simulink model "mySimNN"  (R2021a)
settings: Solver=VariableStepAuto  StartTime=0.0  StopTime=30  MaxStep=1e-3  RelTol=1e-3  EnableMultiTasking=on
values from neighbouring files (symbols this model uses):
  K2 = place(A2, B2, eigs)    [linearizedController.m]
undefined symbols (not defined in the file or in its folder): sigbuilder_block
libraries: simulink x2, deeplib x1
settings Model: Creator=The MathWorks, Inc.  LastModifiedBy=danielpusicha
settings SolverCC: AlgebraicLoopSolver=LineSearch  MinimalZcImpactIntegration=on
settings DataIOCC: LimitDataPoints=on  SaveFormat=Structure  ReturnWorkspaceOutputs=off
settings OptimizationCC: LifeSpan=inf
settings DebuggingCC: AlgebraicLoopMsg=none  UnderspecifiedInitializationDetection=Classic  MergeDetectMultiDrivingBlocksExec=none  SolverPrmCheckMsg=warning  AllowSymbolicDim=off  StateNameClashWarn=warning  SFUnexpectedBacktrackingDiag=warning  SFNoUnconditionalDefaultTransitionDiag=warning  SFExecutionAtInitializationDiag=none  SFMachineParentedDataDiag=warning  ArithmeticOperatorsInVariantConditions=warning
settings HardwareCC: ProdBitPerPointer=32  ProdBitPerSizeT=32  ProdBitPerPtrDiffT=32  ProdLargestAtomicFloat=None  ProdIntDivRoundTo=Undefined  ProdEndianess=Unspecified  ProdWordSize=32  ProdHWDeviceType=32-bit Generic
settings ModelReferenceCC: PropagateSignalLabelsOutOfModel=off
settings SFSimCC: SimUseLocalCustomCode=off  CustomCodeUndefinedFunction=UseInterfaceOnly
settings RTWCC: RTWUseLocalCustomCode=off
settings CodeAppCC: StateflowObjectComments=on
settings GRTTargetCC: TargetLangStandard=C89/C90 (ANSI)
settings ConfigComp: CovMetricSettings=dw  CovSaveCumulativeToWorkspaceVar=on  CovSaveSingleToWorkspaceVar=on  CovExternalEMLEnable=off  CovSFcnEnable=off
settings SimscapeCC: SimscapeNormalizeSystem=off
settings ConfigurationSet: Description=SimMechanics 2G
settings ExplorerConfigSet: InternalSimMechanicsExplorerSettings="<ExplorerConfiguration><canonicalview>default</canonicalview><AnimationSetting><BasePlaybackSpeed>1.0</BasePlaybackSpeed><PlaybackSpeedFactor>1.0</PlaybackSpeedFactor></AnimationSetting><TilePanel><TileInfo><Tiles Columns=\"1\" Count=\"1\" Rows=\"1\"><Column Left=\"2\" Weight=\"1\"/><Column Left=\"1552\"/><Row Top=\"2\" Weight=\"1\"/><Row Top=\"932\"/><Tile Height=\"1\" Width=\"1\" X=\"0\" Y=\"0\"/></Tiles></TileInfo><SceneInfo><SceneViewer><BGColor><R>0.60000002384185791</R><G>0.60000002384185791</G><B>0.60000002384185791</B></BGColor><Camera><Position><X>0.027865189060748197</X><Y>-2.5719092456962986</Y><Z>0.23157896538506753</Z></Position><Center><X>0.62659712312732463</X><Y>-0.46110119691712204</Y><Z>0.22087365386473376</Z></Center><Up><X>-0.0079438354874226333</X><Y>0.0073246425924307582</Y><Z>0.99994162084025784</Z></Up><Left>-0.24533778208815546</Left><Right>0.24533778208815546</Right><Bottom>-0.79734779727023208</Bottom><Top>0.79734779727023208</Top></Camera></SceneViewer></SceneInfo></TilePanel></ExplorerConfiguration>"

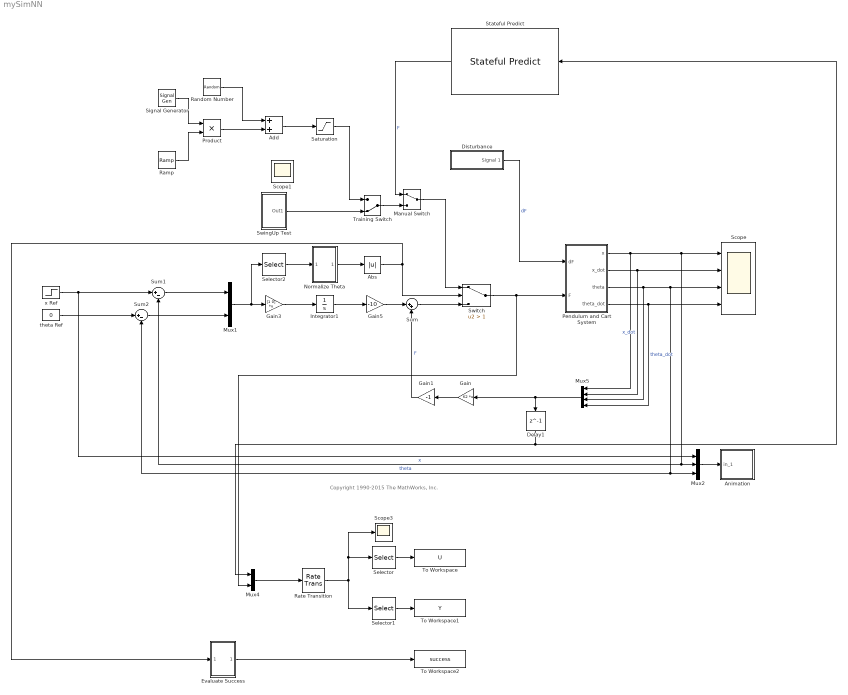
== system mySimNN ==
  note: Copyright 1990-2015 The MathWorks, Inc.
  Abs : Abs
  Add : Sum
  Animation : Subsystem  mask(Pendulum plot){RefBlock=x Ref}
      mask prompts: RefBlock "Cart Reference Signal Block Name:"
      mask help: Pendulum plot
      mask Help: Pendulum animation function using Handle graphics.
      mask Display: plot([-10 10],[0 0],[-2 -2 2 2],[0 1 1 0],[0 3],[1 5])
  Delay1 : Delay  DelayLength=1  SampleTime=0.01
  Disturbance : Subsystem  Tag=STV Subsys  LoadFcn=sigbuilder_block('load');  StartFcn=sigbuilder_block('start');  StopFcn=sigbuilder_block('stop');  ClipboardFcn=sigbuilder_block('clipboard');  mask(Sigbuilder block){tuvar=[0:10]}
      mask help: Simulink:masks:SigbuilderBlock_MD
      mask init:
      | if ~strcmp(get_param(bdroot(gcbh),'SimulationStatus'),'stopped') tuvar = sigbuilder_block('maskInit'); end
      settings: CopyFcn=sigbuilder_block('copy');  DeleteFcn=sigbuilder_block('delete');  ModelCloseFcn=sigbuilder_block('modelClose');  PreSaveFcn=sigbuilder_block('preSave');  PauseFcn=sigbuilder_block('pause');  ContinueFcn=sigbuilder_block('continue');  NameChangeFcn=sigbuilder_block('namechange');  OpenFcn=sigbuilder_block('open',[402.828 199.862 551.172 395.379 ]);  CloseFcn=sigbuilder_block('close');
      mask Display: plot(0, 0, 100, 100,[2, 2, 32, 32, 2], [68, 8, 8, 68, 68],[32, 2], [38, 38], [32, 19, 2],[53, 60, 44], [32, 17, 17, 2],[16, 16, 31, 31]);txt = getActiveGroup(gcbh);text(2, 100, txt,'verticalAlignment', 'top');
  Evaluate Success : Subsystem
  Gain : Gain  Gain=K2  Multiplication=Matrix(K*u)
  Gain1 : Gain  Gain=-1
  Gain3 : Gain  Gain=[1 0]  Multiplication=Matrix(K*u)
  Gain5 : Gain  Gain=-10
  Integrator1 : Integrator
  Manual Switch : ManualSwitch
  Mux1 : Mux  Inputs=2
  Mux2 : Mux  Inputs=3
  Mux4 : Mux  Inputs=2
  Mux5 : Mux
  Normalize Theta : Subsystem
  Pendulum and Cart System : Subsystem  mask{mCartPara=1, mPendPara=1, gPara=9.81, LPara=0.5, KdPara=10}
      mask prompts: mCartPara "Mass of Cart"; mPendPara "Mass of Pendulum"; gPara "Gravity"; LPara "Length of Pendulum"; KdPara "Friction coefficient of Cart"
      mask help: Pendulum and Cart System
      mask init:
      | mCart = str2double(get_param(gcb,'mCartPara'));
      | mPend = str2double(get_param(gcb,'mPendPara'));
      | g = str2double(get_param(gcb,'gPara'));
      | L = str2double(get_param(gcb,'LPara'));
      | Kd = str2double(get_param(gcb,'KdPara'));
  Product : Product
  Ramp : simulink/Sources/Ramp  slope=1  start=0  InitialOutput=0
  Random Number : RandomNumber  Variance=0.1  Seed=533  SampleTime=0.1
  Rate Transition : RateTransition  OutPortSampleTime=.01
  Saturation : Saturate  UpperLimit=50  LowerLimit=-50
  Scope : Scope  NumInputPorts=4
  Scope3 : Scope
  Selector : Selector  InputPortWidth=5  IndexOptions=Index vector (dialog)  Indices=[1: 4]  OutputSizes=1
  Selector1 : Selector  InputPortWidth=5  IndexOptions=Index vector (dialog)  Indices=[ 5]  OutputSizes=1
  Selector2 : Selector  InputPortWidth=2  IndexOptions=Index vector (dialog)  Indices=2  OutputSizes=1
  Signal Generator : SignalGenerator  Amplitude=3  Frequency=4.5  Units=rad/sec
  Stateful Predict : deeplib/Stateful Predict  Network=Network from MAT-file  NetworkFunction=untitled  NetworkFilePath=/Users/danielpusicha/Library/Mobile Documents/com~apple~CloudDocs/Documents/Unterlagen/Studium/Master/Regelungstechnik/Seminararbeit/Simulation/Pendulum On Cart Partially Known/FirstWorkingTrainedNet.mat  InputDataFormats={ '', '' }  SampleTime=-1  ForceInterpretedSim=off  EnableDLNetwork=on
      settings: SourceProductBaseCode=NN
  Sum : Sum  Inputs=|++
  Sum1 : Sum  Inputs=|+-
  Sum2 : Sum  Inputs=|+-
  SwingUp Test : Subsystem
  Switch : Switch  Criteria=u2 > Threshold  Threshold=1
  To Workspace : ToWorkspace  VariableName=U  SampleTime=-1
      settings: Save2DSignal=2-D array (concatenate along first dimension)
  To Workspace1 : ToWorkspace  VariableName=Y  SampleTime=-1
      settings: Save2DSignal=2-D array (concatenate along first dimension)
  To Workspace2 : ToWorkspace  VariableName=success  SampleTime=-1
  Training Switch : ManualSwitch  CurrentSetting=0
  theta Ref : Constant  Value=0
  x Ref : Step  After=10  SampleTime=0
  Scope1 : Scope
  wires:
  Pendulum and Cart System/4(theta_dot) -> Mux5/4, Scope/4  "theta_dot"
  Pendulum and Cart System/3(theta) -> Mux5/3, Sum2/2, Mux2/3, Scope/3  "theta"
  Pendulum and Cart System/2(x_dot) -> Mux5/2, Scope/2  "x_dot"
  Pendulum and Cart System/1(x) -> Mux5/1, Sum1/2, Mux2/2, Scope/1  "x"
  Disturbance/1(Signal 1) -> Pendulum and Cart System/1(dF)  "dF"
  Gain1/1 -> Sum/2  "F"
  Mux2/1 -> Animation/1(in_1)
  x Ref/1 -> Mux2/1, Sum1/1
  Mux4/1 -> Rate Transition/1
  Selector/1 -> To Workspace/1
  Selector1/1 -> To Workspace1/1
  Rate Transition/1 -> Scope3/1, Selector/1, Selector1/1
  Switch/1 -> Pendulum and Cart System/2(F), Mux4/2
  theta Ref/1 -> Sum2/1
  Gain/1 -> Gain1/1
  Mux1/1 -> Selector2/1, Gain3/1
  Gain3/1 -> Integrator1/1
  Integrator1/1 -> Gain5/1
  Gain5/1 -> Sum/1
  Sum1/1 -> Mux1/1
  Sum2/1 -> Mux1/2
  Selector2/1 -> Normalize Theta/1(In1)
  Normalize Theta/1(Out1) -> Abs/1
  Sum/1 -> Switch/3
  Manual Switch/1 -> Switch/1
  SwingUp Test/1(Out1) -> Training Switch/2
  Signal Generator/1 -> Product/1
  Saturation/1 -> Training Switch/1
  Ramp/1 -> Product/2
  Abs/1 -> Switch/2, Evaluate Success/1(In1)
  Evaluate Success/1(Out1) -> To Workspace2/1
  Product/1 -> Add/2
  Random Number/1 -> Add/1
  Add/1 -> Saturation/1
  Training Switch/1 -> Manual Switch/2
  Stateful Predict/1 -> Manual Switch/1  "F"
  Mux5/1 -> Gain/1, Delay1/1
  Delay1/1 -> Stateful Predict/1, Mux4/1

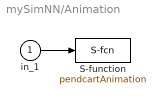
== system mySimNN/Animation ==
  in_1 : Inport
  S-function : S-Function  FunctionName=pendcartAnimation  Parameters=RefBlock  SFunctionDeploymentMode=off  EnableBusSupport=off
      settings: DeleteFcn=pendcartAnimation([],[],[],'DeleteBlock');
  wires:
  in_1/1 -> S-function/1

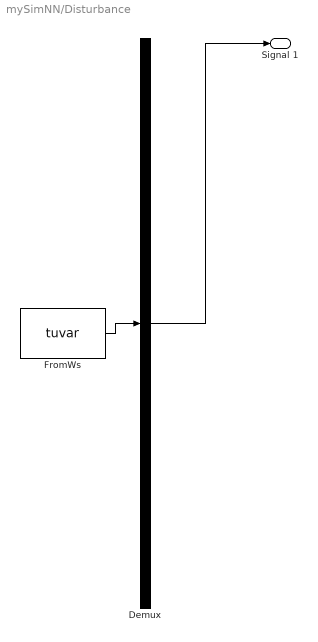
== system mySimNN/Disturbance ==
  Demux : Demux  Tag=STV Demux  Outputs=1
      settings: DisplayOption=none
  FromWs : FromWorkspace  Tag=STV FromWs  VariableName=tuvar
      SigBuilderData=|
      | common.afterFinalStr = 'Extrapolate'
      | common.sampleTime = 0
      | dataSet.timeRange = [0 20]
      | dataSet.name = 'Group 1'
      | sbobj.Groups.Name = 'Group 1'
      | sbobj.Groups.Signals.Name = 'Signal 1'
      | sbobj.Groups.Signals.XData = [0 15 15.5 16 20]
      | sbobj.Groups.Signals.YData = [0 0 2 0 0]
      | sbobj.Groups.TimeRange = [0 20]
  Signal 1 : Outport  Tag=STV Outport  VectorParamsAs1DForOutWhenUnconnected=off
  wires:
  FromWs/1 -> Demux/1
  Demux/1 -> Signal 1/1

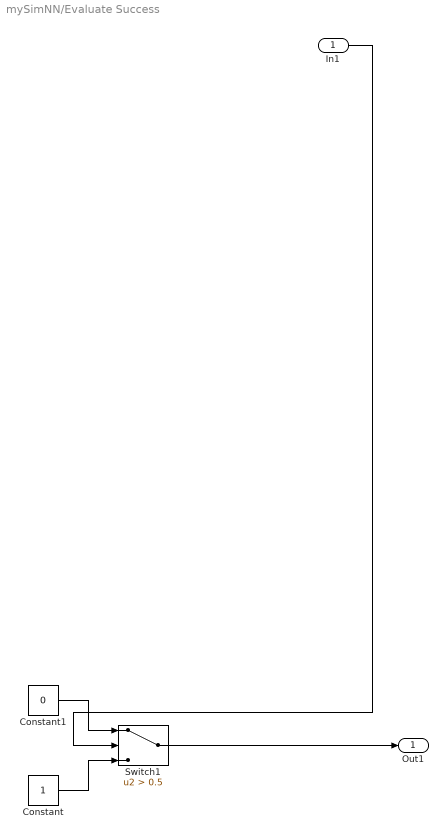
== system mySimNN/Evaluate Success ==
  In1 : Inport
  Constant : Constant
  Constant1 : Constant  Value=0
  Switch1 : Switch  Criteria=u2 > Threshold  Threshold=0.5
  Out1 : Outport
  wires:
  Switch1/1 -> Out1/1
  In1/1 -> Switch1/2
  Constant1/1 -> Switch1/1
  Constant/1 -> Switch1/3

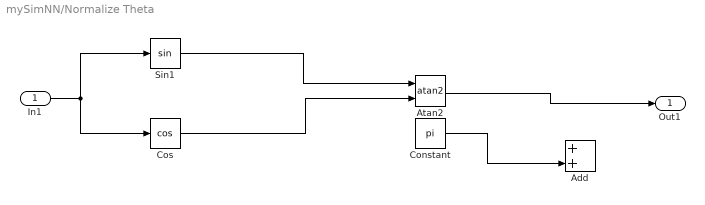
== system mySimNN/Normalize Theta ==
  In1 : Inport
  Add : Sum
  Atan2 : Trigonometry  Operator=atan2
  Constant : Constant  Value=pi
  Cos : Trigonometry  Operator=cos
  Sin1 : Trigonometry
  Out1 : Outport
  wires:
  In1/1 -> Cos/1, Sin1/1
  Sin1/1 -> Atan2/1
  Cos/1 -> Atan2/2
  Atan2/1 -> Out1/1
  Constant/1 -> Add/2

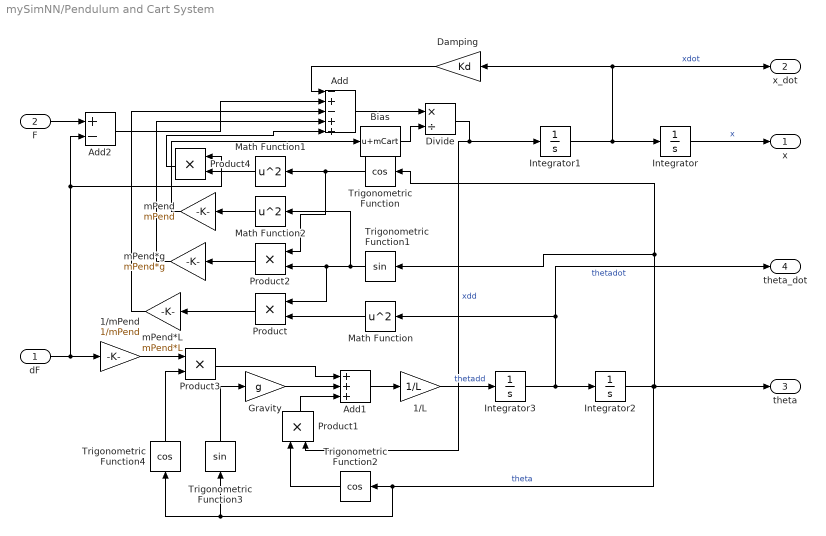
== system mySimNN/Pendulum and Cart System ==
  dF : Inport
  F : Inport  Port=2
  1/L : Gain  Gain=1/L
  1/mPend : Gain  Gain=1/mPend
  Add : Sum  Inputs=-+-++
  Add1 : Sum  Inputs=+++
  Add2 : Sum  Inputs=+-
  Bias : Bias  Bias=mCart
  Damping : Gain  Gain=Kd
  Divide : Product  Inputs=*/
  Gravity : Gain  Gain=g
  Integrator : Integrator  ContinuousStateAttributes='x'
  Integrator1 : Integrator  ContinuousStateAttributes='xdot'
  Integrator2 : Integrator  InitialCondition=pi  ContinuousStateAttributes='theta'
  Integrator3 : Integrator  ContinuousStateAttributes='thetadot'
  Math Function : Math  Operator=square  SignedPower=on  SaturateOnIntegerOverflow=on
  Math Function1 : Math  Operator=square  SignedPower=on  SaturateOnIntegerOverflow=on
  Math Function2 : Math  Operator=square  SignedPower=on  SaturateOnIntegerOverflow=on
  Product{,1..4} (5 alike) : Product
  Trigonometric Function : Trigonometry  Operator=cos
  Trigonometric Function1 : Trigonometry
  Trigonometric Function2 : Trigonometry  Operator=cos
  Trigonometric Function3 : Trigonometry
  Trigonometric Function4 : Trigonometry  Operator=cos
  mPend : Gain  Gain=mPend
  mPend*L : Gain  Gain=mPend*L
  mPend*g : Gain  Gain=mPend*g
  x : Outport  VectorParamsAs1DForOutWhenUnconnected=off
  x_dot : Outport  Port=2  VectorParamsAs1DForOutWhenUnconnected=off
  theta : Outport  Port=3  VectorParamsAs1DForOutWhenUnconnected=off
  theta_dot : Outport  Port=4  VectorParamsAs1DForOutWhenUnconnected=off
  wires:
  mPend/1 -> Bias/1
  Bias/1 -> Divide/2
  Math Function2/1 -> mPend/1
  Product4/1 -> Add/5
  Math Function1/1 -> Product4/2
  mPend*g/1 -> Add/4
  Product1/1 -> Add1/3
  Math Function/1 -> Product/2
  1/L/1 -> Integrator3/1  "thetadd"
  dF/1 -> 1/mPend/1, Product4/1, Add2/2
  1/mPend/1 -> Product3/1
  Trigonometric Function4/1 -> Product3/2
  Damping/1 -> Add/1
  F/1 -> Add2/1
  Trigonometric Function3/1 -> Gravity/1
  Gravity/1 -> Add1/2
  Trigonometric Function/1 -> Math Function1/1, Product2/1
  Integrator3/1 -> Integrator2/1, Math Function/1, theta_dot/1  "thetadot"
  Integrator2/1 -> Trigonometric Function2/1, Trigonometric Function3/1, Trigonometric Function4/1, Trigonometric Function1/1, Trigonometric Function/1, theta/1  "theta"
  Product3/1 -> Add1/1
  Add/1 -> Divide/1
  Divide/1 -> Integrator1/1, Product1/2  "xdd"
  Trigonometric Function2/1 -> Product1/1
  Trigonometric Function1/1 -> Math Function2/1, Product/1, Product2/2
  Integrator/1 -> x/1  "x"
  Integrator1/1 -> Damping/1, x_dot/1, Integrator/1  "xdot"
  Product2/1 -> mPend*g/1
  Add1/1 -> 1/L/1
  Add2/1 -> Add/2
  mPend*L/1 -> Add/3
  Product/1 -> mPend*L/1

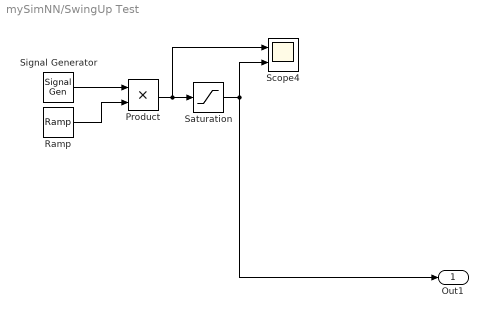
== system mySimNN/SwingUp Test ==
  Product : Product
  Ramp : simulink/Sources/Ramp  slope=1  start=0  InitialOutput=0
  Saturation : Saturate  UpperLimit=50  LowerLimit=-50
  Scope4 : Scope  NumInputPorts=2
  Signal Generator : SignalGenerator  Amplitude=3  Frequency=4.5  Units=rad/sec
  Out1 : Outport
  wires:
  Product/1 -> Scope4/1, Saturation/1
  Ramp/1 -> Product/2
  Signal Generator/1 -> Product/1
  Saturation/1 -> Out1/1, Scope4/2
